simulink model "dof1_system"  (R2024b)
settings: Solver=ode3  StartTime=0.0  StopTime=100  FixedStep=0.01  RelTol=1e-3
values from neighbouring files (symbols this model uses):
  k = (rho * C_X * A) / (m_t * 2)    (= 0.000199261761762)    [braking_dist.m]
undefined symbols (not defined in the file or in its folder): c, dq0, M, q0
settings Model: Creator=martinhaugen  LastModifiedBy=martinhaugen

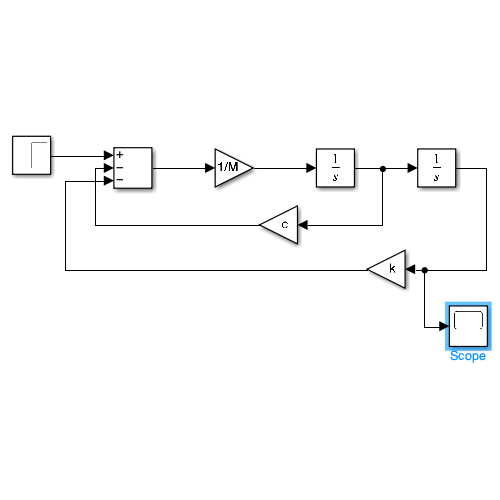
[thumbnail: Simulink's stored preview of the top-level diagram]
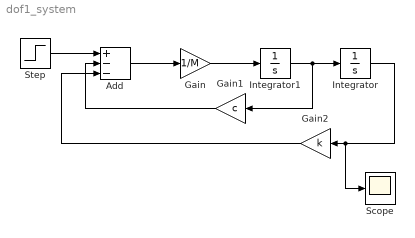
== system dof1_system ==
  Add : Sum  Inputs=+--
  Gain : Gain  Gain=1/M
  Gain1 : Gain  Gain=c
  Gain2 : Gain  Gain=k
  Integrator : Integrator  InitialCondition=q0
  Integrator1 : Integrator  InitialCondition=dq0
  Scope : Scope
  Step : Step  SampleTime=0
  wires:
  Add/1 -> Gain/1
  Gain/1 -> Integrator1/1
  Integrator1/1 -> Gain1/1, Integrator/1
  Gain1/1 -> Add/2
  Integrator/1 -> Scope/1, Gain2/1
  Gain2/1 -> Add/3
  Step/1 -> Add/1
